simulink model "GMSK_Rayleigh"  (R2020b)
settings: Solver=VariableStepAuto  StartTime=0.0  StopTime=1e-1  RelTol=1e-3
undefined symbols (not defined in the file or in its folder): doppler
libraries: commutil2 x3, commchan3 x2, commdigbbndcpm2 x2, commfilt2 x2, commsink2 x1, commrandsrc3 x1, dspstat3 x1
settings Model: Creator=giusp  LastModifiedBy=giusp

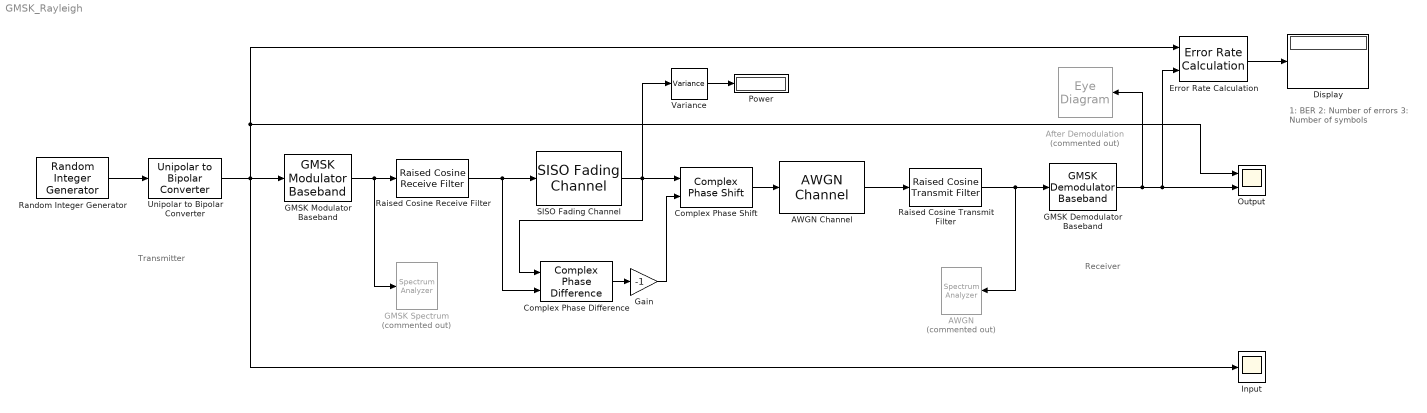
== system GMSK_Rayleigh ==
  note: Transmitter
  note: Receiver
  note: 1: BER
      | 2: Number of errors
      | 3: Number of symbols
  AWGN : SpectrumAnalyzer  Commented=on
  AWGN Channel : commchan3/AWGN Channel  InputProcessing=Columns as channels (frame based)  seed=67  noiseMode="Signal to noise ratio  (Eb/No)"  EbNodB=-2  EsNodB=10  SNRdB=10  bitsPerSym=1  Ps=8.2  Tsym=1e-6  variance=1
  After Demodulation : EyeDiagram  Commented=on
  Complex Phase Difference : commutil2/Complex Phase Difference
      settings: SourceProductBaseCode=CM
  Complex Phase Shift : commutil2/Complex Phase Shift
      settings: SourceProductBaseCode=CM
  Display : Display
  Error Rate Calculation : commsink2/Error Rate Calculation  N=26  st_delay=0  cp_mode=Entire frame  subframe=[]  PMode=Port  WsName=ErrorVec  RsMode2=off  stop=off  numErr=100  maxBits=1e6
  GMSK Demodulator Baseband : commdigbbndcpm2/GMSK Demodulator Baseband  OutputType=Integer  BT=.3  pulseLength=4  preHistory=1  phaseOffset=0  samplesPerSymbol=4  RateOptions=Enforce single-rate processing  traceBack=16  outDType=double
      settings: SourceProductBaseCode=CM
  GMSK Modulator Baseband : commdigbbndcpm2/GMSK Modulator Baseband  inputType=Integer  BT=.3  pulseLength=4  preHistory=1  phaseOffset=0  samplesPerSymbol=4  RateOptions=Enforce single-rate processing  outDataType=double
      settings: SourceProductBaseCode=CM
  GMSK Spectrum : SpectrumAnalyzer  Commented=on
  Gain : Gain  Gain=-1
  Input : Scope
  Output : Scope  NumInputPorts=2
  Power : Display
  Raised Cosine Receive Filter : commfilt2/Raised Cosine Receive Filter  filtType=Square root  R=0.2  filtSpan=10  N=4  downFactor=4  downOffset=0  filterGain=1  InputProcessing=Columns as channels (frame based)  RateOptions=Enforce single-rate processing  framing=Mute  checkCoeff=off  variableName=rcRxFilt  currentFiltSpan=10  D=5  inputOffset=0  sampMode=Mute  saveAsFlag=0  rateMode=Downsampling  checkGain=Normalized  launchFVT=on  roundingMode=Floor  overflowMode=off  coeffDataTypeStr=Inherit: Same word length as input  coeffMin=[]  coeffMax=[]  coeffLastDataTypeStr=Inherit: Same word length as input  accumDataTypeStr=Inherit: Same as product output  accumLastDataTypeStr=Inherit: Same as product output  outputDataTypeStr=Inherit: Same as accumulator  outputMin=[]  outputMax=[]  outputLastDataTypeStr=Inherit: Same as accumulator
  Raised Cosine Transmit Filter : commfilt2/Raised Cosine Transmit Filter  filtType=Square root  R=0.2  filtSpan=10  N=4  filterGain=1  InputProcessing=Columns as channels (frame based)  RateOptions=Enforce single-rate processing  framing=Mute  checkCoeff=off  variableName=rcTxFilt  checkGain=Normalized  sampMode=Mute  saveAsFlag=0  currentFiltSpan=10  D=(10)/2  launchFVT=on  roundingMode=Floor  overflowMode=off  coeffDataTypeStr=Inherit: Same word length as input  coeffMin=[]  coeffMax=[]  coeffLastDataTypeStr=Inherit: Same word length as input  outputDataTypeStr=Inherit: Same as accumulator  outputMin=[]  outputMax=[]  outputLastDataTypeStr=Inherit: Same as accumulator
  Random Integer Generator : commrandsrc3/Random Integer Generator  SetSize=2  SeedSource=Auto  Seed=0  SampleTime=1e-6  SamplesPerFrame=1  OutputDataType=double  SimulateUsing=Interpreted execution
  SISO Fading Channel : commchan3/SISO Fading Channel  InheritSampleRate=on  SampleRate=1  PathDelays=1e-5*[0.2 0.4 0.6]  AveragePathGains=[0 -3 -6]  NormalizePathGains=on  FadingDistribution=Rayleigh  KFactor=3  DirectPathDopplerShift=0  DirectPathInitialPhase=0  MaximumDopplerShift=0.001  DopplerSpectrum=doppler('Jakes')  RandomStream=mt19937ar with seed  Seed=73  PathGainsOutputPort=off  ChannelFilterDelayOutputPort=off  SimulateUsing=Interpreted execution  Visualization=Off  PathsForDopplerDisplay=1  SamplesToDisplay=50%
  Unipolar to Bipolar Converter : commutil2/Unipolar to Bipolar Converter  M=2  polarity=Positive  dataType=Inherit via internal rule
  Variance : dspstat3/Variance  run=on  InputProcessing=Columns as channels (frame based)  reset_popup=None  directionMode=Each column  dimension=1  roiEnable=off  roiType=Rectangles  roiPortion=Entire ROI  roiOutput=Individual statistics for each ROI  roiFlag=off  roundingMode=Floor  overflowMode=off
  wires:
  GMSK Modulator Baseband/1 -> Raised Cosine Receive Filter/1, GMSK Spectrum/1
  Random Integer Generator/1 -> Unipolar to Bipolar Converter/1
  GMSK Demodulator Baseband/1 -> After Demodulation/1, Output/2, Error Rate Calculation/2
  Unipolar to Bipolar Converter/1 -> GMSK Modulator Baseband/1, Output/1, Error Rate Calculation/1, Input/1
  Raised Cosine Transmit Filter/1 -> GMSK Demodulator Baseband/1, AWGN/1
  Error Rate Calculation/1 -> Display/1
  Raised Cosine Receive Filter/1 -> Complex Phase Difference/2, SISO Fading Channel/1
  Variance/1 -> Power/1
  SISO Fading Channel/1 -> Complex Phase Shift/1, Complex Phase Difference/1, Variance/1
  AWGN Channel/1 -> Raised Cosine Transmit Filter/1
  Complex Phase Difference/1 -> Gain/1
  Gain/1 -> Complex Phase Shift/2
  Complex Phase Shift/1 -> AWGN Channel/1
